simulink model "sensores"  (R2022b)
settings: Solver=VariableStepAuto  StartTime=0.0  StopTime=10.0  RelTol=1e-3
libraries: arduinolib x2
settings Model: Creator=alber  LastModifiedBy=alber

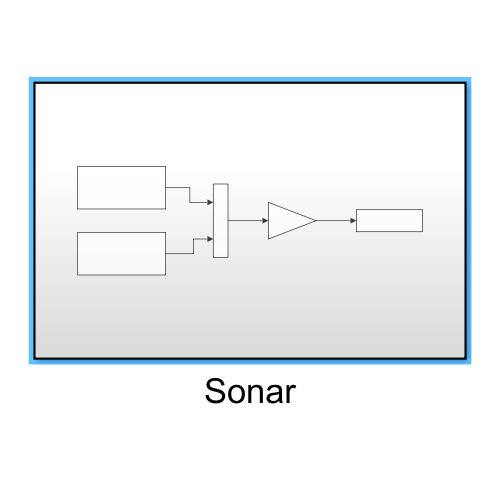
[thumbnail: Simulink's stored preview of the top-level diagram]
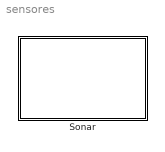
== system sensores ==
  Sonar : Subsystem

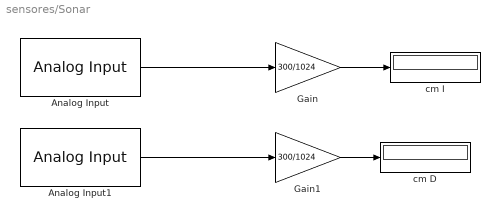
== system sensores/Sonar ==
  Analog Input : arduinolib/Analog Input  pinNumber=4  ReadResultsOnly=off  ConversionTriggerSource=Software  ExternalTriggerType=uint32( 0 )  OutputDataType=uint16  EnableConversionCompleteNotify=off  EnableOuputStatus=off  SampleTime=-1  blockPlatform=arduino
  Analog Input1 : arduinolib/Analog Input  pinNumber=5  ReadResultsOnly=off  ConversionTriggerSource=Software  ExternalTriggerType=uint32( 0 )  OutputDataType=uint16  EnableConversionCompleteNotify=off  EnableOuputStatus=off  SampleTime=-1  blockPlatform=arduino
  Gain : Gain  Gain=300/1024
  Gain1 : Gain  Gain=300/1024
  cm D : Display
  cm I : Display
  wires:
  Analog Input/1 -> Gain/1
  Gain/1 -> cm I/1
  Analog Input1/1 -> Gain1/1
  Gain1/1 -> cm D/1
